simulink library "ude"  (Simulink 8.2)
settings: Solver=ode1  StartTime=0.0  StopTime=Inf  FixedStep=0.001  RelTol=1e-3
PostLoadFcn:
  | , if any(exist('dsrtsu_mdlpostloadfcn', 'file') == [2, 3, 6]), try dsrtsu_mdlpostloadfcn('Execute', bdroot); catch fprintf('Error in PostLoadFcn (dsrtsu_mdlpostloadfcn) for model "%s":\n %s\n', bdroot, lasterr); end, end,
undefined symbols (not defined in the file or in its folder): FALSE, TRUE
libraries: hcu_lib x4, simulink x2
(part 1 of 2)
settings Model: RequirementInfo="{}  %GIDa_987fab82_ea26_42c4_899d_f6cf30f28fd4"  DSRTSU_INTERNAL_RTI_VER=450  DSRTSU_INTERNAL_RTI_TYPE=rti1401  RTICANMMDATA=struct('GeneralSetupData',struct('modelroot','D:\ActiveSafetyDepartment\SVN\trunk\ADAS_Softwares\HTDragon\software\sw_development\arch\app\ude','generalsettings',struct('filesettings',struct('destfolder',struct('Name','RTICANMM_FILES','Check',1),'buildfolder',struct('Name','.','Check',1),'AbsDestfolder',struct('Name','D:\ActiveSafetyDepartment\SVN\trunk\ADAS_Softwares\HTDragon\software\sw_development\arch\app\ude\RTICANMM_FILES'),'AbsBuildfolder',struct('Name','D:\ActiveSafetyDepartment\SVN\trunk\ADAS_Softwares\HTDragon\software\sw_development\arch\app\ude'))),'options',struct('addpaths',1,'rmpaths',1,'addtrcexclusion',logical(1),'cannavigator',struct('checkmonitoring',0),'show_usrtrc',0,'use_usrtrc',0),'advanced',struct('options',[1 1 1 1 1 1 1 1 1 1 1 1 1 1 1 1 1 1 1 1 1 1 1 1 1 1 1 1 1 1 1 1 1 1 1 1 1 1 1 1 1 1 1 1 1 1 1 1 1 1 1 1 1 1 1 1 1 1 1 1 1 1 1 1 1 1 1 1 1 1 1 1 1 1 1 1 1 1 1 1 1 1 1 1 1 1 1 1 1 1 1 1 1 1 1 1 1 1 1 1]),'MPSetup',{{}},'modelname','ude','block','ude'))  DSRTSU_INTERNAL_RTIFPGA=40  Creator=11116  LastModifiedBy=14069

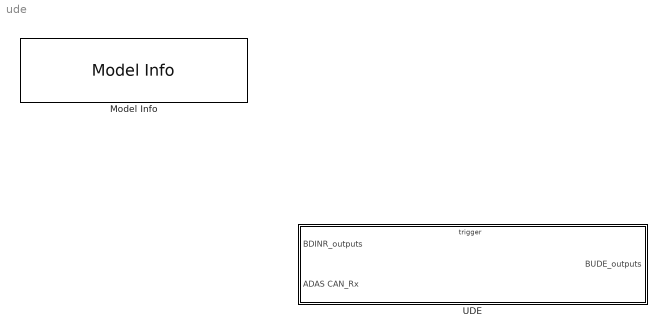
== system ude ==
  Model Info : simulink/Model-Wide Utilities/Model Info  InitialBlockCM=None  BlockCM=None  Frame=on  DisplayStringWithTags=|  HorizontalTextAlignment=Left  LeftAlignmentValue=0.02  SourceBlockDiagram=ude  TagMaxNumber=20
      | Model Version        : %<ModelVersion>
      | Creator                   : %<Creator>
      | Last Modified By    : %<LastModifiedBy>
  UDE : Subsystem
      settings: RTWSystemCode=Nonreusable function  RTWFcnNameOpts=Use subsystem name  RTWFileNameOpts=Use subsystem name

== system ude/UDE ==
  BDINR_outputs : Inport  OutDataTypeStr=Bus: BDINR_outputs
  ADAS CAN_Rx : Inport  Port=2
  trig_UDE : TriggerPort  TriggerType=function-call
  ude : Subsystem
  BUDE_outputs : Outport
  wires:
  ADAS CAN_Rx/1 -> ude/2(ADAS CAN_Rx)
  BDINR_outputs/1 -> ude/1(BDINR_outputs)
  ude/1(BUDE_outputs) -> BUDE_outputs/1

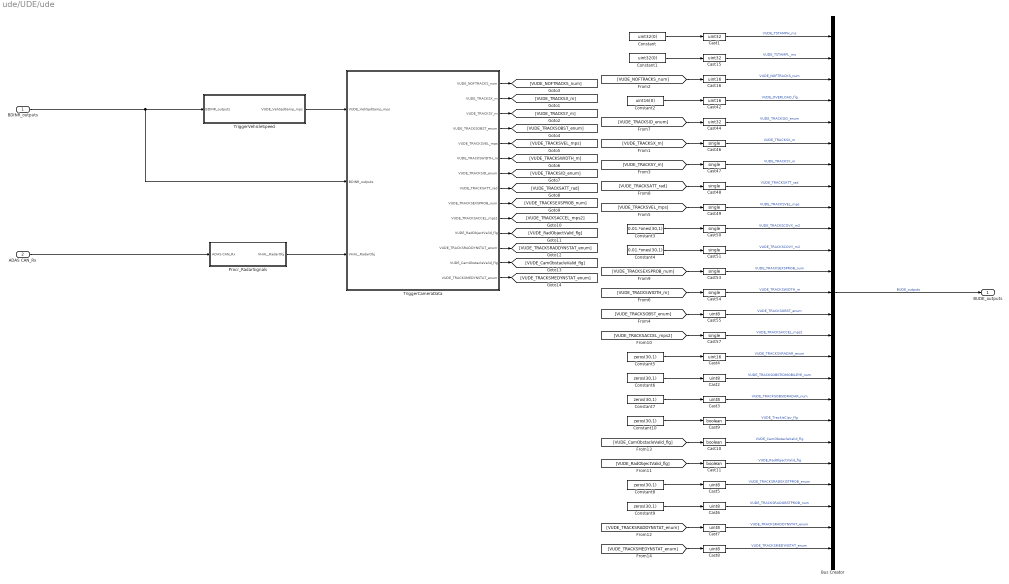
== system ude/UDE/ude ==
  BDINR_outputs : Inport
  ADAS CAN_Rx : Inport  Port=2
  Bus Creator : BusCreator  Inputs=25  OutDataTypeStr=Bus: BUDE_outputs
  Cast1 : DataTypeConversion  OutDataTypeStr=uint32  RndMeth=Zero
  Cast10 : DataTypeConversion  OutDataTypeStr=boolean  RndMeth=Zero
  Cast11 : DataTypeConversion  OutDataTypeStr=boolean  RndMeth=Zero
  Cast15 : DataTypeConversion  OutDataTypeStr=uint32  RndMeth=Zero
  Cast16 : DataTypeConversion  OutDataTypeStr=uint16  RndMeth=Zero
  Cast{2..3,5..8,55} (7 alike) : DataTypeConversion  OutDataTypeStr=uint8  RndMeth=Zero
  Cast4 : DataTypeConversion  OutDataTypeStr=uint16  RndMeth=Zero
  Cast42 : DataTypeConversion  OutDataTypeStr=uint16  RndMeth=Zero
  Cast44 : DataTypeConversion  OutDataTypeStr=uint32  RndMeth=Zero
  Cast{46..51,53..54,57} (9 alike) : DataTypeConversion  OutDataTypeStr=single  RndMeth=Zero
  Cast9 : DataTypeConversion  OutDataTypeStr=boolean  RndMeth=Zero
  Constant : Constant  Value=uint32(0)
  Constant1 : Constant  Value=uint32(0)
  Constant10 : Constant  Value=zeros(30,1)  OutDataTypeStr=boolean
  Constant2 : Constant  Value=uint16(0)
  Constant3 : Constant  Value=0.01.*ones(30,1)  OutDataTypeStr=single
  Constant4 : Constant  Value=0.01.*ones(30,1)  OutDataTypeStr=single
  Constant5 : Constant  Value=zeros(30,1)  OutDataTypeStr=uint16
  Constant{6..9} (4 alike) : Constant  Value=zeros(30,1)  OutDataTypeStr=uint8
  Procr_RadarSignals : Subsystem
  TriggerCameraData : Subsystem  TreatAsAtomicUnit=on
  TriggerVehicleSpeed : Subsystem  TreatAsAtomicUnit=on
  BUDE_outputs : Outport  OutDataTypeStr=Bus: BUDE_outputs
  wires:
  Constant9/1 -> Cast6/1
  Constant8/1 -> Cast5/1
  Constant7/1 -> Cast3/1
  Constant6/1 -> Cast2/1
  Constant5/1 -> Cast4/1
  Constant10/1 -> Cast9/1
  Constant4/1 -> Cast51/1
  Constant3/1 -> Cast50/1
  Constant2/1 -> Cast42/1
  [VUDE_CamObstacleValid_flg] -> Cast10/1
  [VUDE_TRACKSMEDYNSTAT_enum] -> Cast8/1
  [VUDE_TRACKSRADDYNSTAT_enum] -> Cast7/1
  [VUDE_RadObjectValid_flg] -> Cast11/1
  [VUDE_TRACKSACCEL_mps2] -> Cast57/1
  [VUDE_TRACKSEXSPROB_num] -> Cast53/1
  [VUDE_TRACKSATT_rad] -> Cast48/1
  [VUDE_TRACKSID_enum] -> Cast44/1
  [VUDE_TRACKSWIDTH_m] -> Cast54/1
  [VUDE_TRACKSVEL_mps] -> Cast49/1
  [VUDE_TRACKSOBST_enum] -> Cast55/1
  [VUDE_TRACKSY_m] -> Cast47/1
  [VUDE_TRACKSX_m] -> Cast46/1
  [VUDE_NOFTRACKS_num] -> Cast16/1
  TriggerCameraData/14(VUDE_TRACKSMEDYNSTAT_enum) -> [VUDE_TRACKSMEDYNSTAT_enum]
  TriggerCameraData/13(VUDE_CamObstacleValid_flg) -> [VUDE_CamObstacleValid_flg]
  TriggerCameraData/12(VUDE_TRACKSRADDYNSTAT_enum) -> [VUDE_TRACKSRADDYNSTAT_enum]
  TriggerCameraData/11(VUDE_RadObjectValid_flg) -> [VUDE_RadObjectValid_flg]
  TriggerCameraData/10(VUDE_TRACKSACCEL_mps2) -> [VUDE_TRACKSACCEL_mps2]
  TriggerCameraData/9(VUDE_TRACKSEXSPROB_num) -> [VUDE_TRACKSEXSPROB_num]
  TriggerCameraData/8(VUDE_TRACKSATT_rad) -> [VUDE_TRACKSATT_rad]
  TriggerCameraData/7(VUDE_TRACKSID_enum) -> [VUDE_TRACKSID_enum]
  TriggerCameraData/6(VUDE_TRACKSWIDTH_m) -> [VUDE_TRACKSWIDTH_m]
  TriggerCameraData/5(VUDE_TRACKSVEL_mps) -> [VUDE_TRACKSVEL_mps]
  TriggerCameraData/4(VUDE_TRACKSOBST_enum) -> [VUDE_TRACKSOBST_enum]
  TriggerCameraData/3(VUDE_TRACKSY_m) -> [VUDE_TRACKSY_m]
  TriggerCameraData/2(VUDE_TRACKSX_m) -> [VUDE_TRACKSX_m]
  TriggerCameraData/1(VUDE_NOFTRACKS_num) -> [VUDE_NOFTRACKS_num]
  Cast8/1 -> Bus Creator/25  "VUDE_TRACKSMEDYNSTAT_enum"
  Cast11/1 -> Bus Creator/21  "VUDE_RadObjectValid_flg"
  Cast10/1 -> Bus Creator/20  "VUDE_CamObstacleValid_flg"
  Cast9/1 -> Bus Creator/19  "VUDE_TrackIsCipv_flg"
  Cast7/1 -> Bus Creator/24  "VUDE_TRACKSRADDYNSTAT_enum"
  Cast6/1 -> Bus Creator/23  "VUDE_TRACKSRADOBSTPROB_num"
  Cast5/1 -> Bus Creator/22  "VUDE_TRACKSRADEXISTPROB_enum"
  Cast3/1 -> Bus Creator/18  "VUDE_TRACKSOBSIDRADAR_num"
  Cast2/1 -> Bus Creator/17  "VUDE_TRACKSOBSTIDMOBILEYE_num"
  Cast53/1 -> Bus Creator/12  "VUDE_TRACKSEXSPROB_num"
  Cast54/1 -> Bus Creator/13  "VUDE_TRACKSWIDTH_m"
  Cast55/1 -> Bus Creator/14  "VUDE_TRACKSOBST_enum"
  Cast57/1 -> Bus Creator/15  "VUDE_TRACKSACCEL_mps2"
  Cast51/1 -> Bus Creator/11  "VUDE_TRACKSCOVY_m2"
  Cast50/1 -> Bus Creator/10  "VUDE_TRACKSCOVX_m2"
  Cast49/1 -> Bus Creator/9  "VUDE_TRACKSVEL_mps"
  Cast48/1 -> Bus Creator/8  "VUDE_TRACKSATT_rad"
  Cast47/1 -> Bus Creator/7  "VUDE_TRACKSY_m"
  Cast46/1 -> Bus Creator/6  "VUDE_TRACKSX_m"
  Cast44/1 -> Bus Creator/5  "VUDE_TRACKSID_enum"
  Cast42/1 -> Bus Creator/4  "VUDE_OVERLOAD_flg"
  Cast16/1 -> Bus Creator/3  "VUDE_NOFTRACKS_num"
  Cast15/1 -> Bus Creator/2  "VUDE_TSTAMPL_ms"
  Cast1/1 -> Bus Creator/1  "VUDE_TSTAMPH_ms"
  Bus Creator/1 -> BUDE_outputs/1  "BUDE_outputs"
  Cast4/1 -> Bus Creator/16  "VUDE_TRACKSVRADAR_enum"
  Constant/1 -> Cast1/1
  Constant1/1 -> Cast15/1
  BDINR_outputs/1 -> TriggerCameraData/2(BDINR_outputs), TriggerVehicleSpeed/1(BDINR_outputs)
  TriggerVehicleSpeed/1(VUDE_VehSpdSamp_mps) -> TriggerCameraData/1(VUDE_VehSpdSamp_mps)
  Procr_RadarSignals/1(VHAL_RadarObj) -> TriggerCameraData/3(VHAL_RadarObj)
  ADAS CAN_Rx/1 -> Procr_RadarSignals/1(ADAS CAN_Rx)

== system ude/UDE/ude/Procr_RadarSignals ==
  ADAS CAN_Rx : Inport
  Bus Creator : BusCreator  Inputs=11
  Procr_RadarSignals : Subsystem
  VHAL_RadarObj : Outport
  wires:
  ADAS CAN_Rx/1 -> Procr_RadarSignals/1(ADAS CAN_Rx)
  Procr_RadarSignals/7(VHAL_RadarObjType10_enum_InProc) -> Bus Creator/7
  Procr_RadarSignals/5(VHAL_RadarObjVelX10_mps_InProc) -> Bus Creator/5
  Procr_RadarSignals/8(VHAL_RadarObjVelY10_mps_InProc) -> Bus Creator/8
  Procr_RadarSignals/3(VHAL_RadarObjPosX10_m_InProc) -> Bus Creator/3
  Procr_RadarSignals/9(VHAL_RadarObjAccX10_mps2_InProc) -> Bus Creator/9
  Procr_RadarSignals/4(VHAL_RadarObjPosY10_m_InProc) -> Bus Creator/4
  Procr_RadarSignals/2(VHAL_RadarObjID10_num_InProc) -> Bus Creator/2
  Procr_RadarSignals/6(VHAL_RadarObjStatus10_enum_InProc) -> Bus Creator/6
  Bus Creator/1 -> VHAL_RadarObj/1
  Procr_RadarSignals/1(VHAL_NoObj_num_InProc) -> Bus Creator/1
  Procr_RadarSignals/10(VHAL_RadarObjValid10_flg_InProc) -> Bus Creator/10
  Procr_RadarSignals/11(VHAL_RadarObjWidth10_m_InProc) -> Bus Creator/11

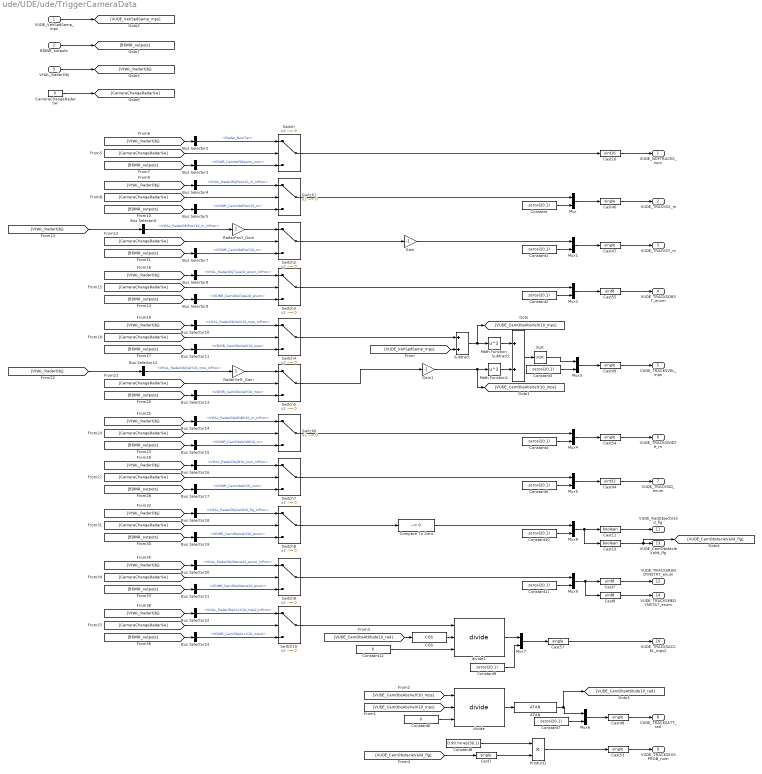
== system ude/UDE/ude/TriggerCameraData ==
  VUDE_VehSpdSamp_mps : Inport
  BDINR_outputs : Inport  Port=2
  VHAL_RadarObj : Inport  Port=3
  ATAN : hcu_lib/ATAN
  Bus Selector10 : BusSelector  OutputSignals=VHAL_RadarObjVelX10_mps_InProc
  Bus Selector11 : BusSelector  OutputSignals=VDINR_CamObsVelX10_mps
  Bus Selector12 : BusSelector  OutputSignals=VHAL_RadarObjVelY10_mps_InProc
  Bus Selector13 : BusSelector  OutputSignals=VDINR_CamObsVelY10_mps
  Bus Selector14 : BusSelector  OutputSignals=VHAL_RadarObjWidth10_m_InProc
  Bus Selector15 : BusSelector  OutputSignals=VDINR_CamObsWidth10_m
  Bus Selector16 : BusSelector  OutputSignals=VHAL_RadarObjID10_num_InProc
  Bus Selector17 : BusSelector  OutputSignals=VDINR_CamObsID10_num
  Bus Selector18 : BusSelector  OutputSignals=VHAL_RadarObjValid10_flg_InProc
  Bus Selector19 : BusSelector  OutputSignals=VDINR_CamObsValid10_enum
  Bus Selector2 : BusSelector  OutputSignals=Radar_NumTar
  Bus Selector20 : BusSelector  OutputSignals=VHAL_RadarObjStatus10_enum_InProc
  Bus Selector21 : BusSelector  OutputSignals=VDINR_CamObsStatus10_enum
  Bus Selector22 : BusSelector  OutputSignals=VHAL_RadarObjAccX10_mps2_InProc
  Bus Selector23 : BusSelector  OutputSignals=VDINR_CamObsAccX10_mps2
  Bus Selector3 : BusSelector  OutputSignals=VDINR_CamNofObjects_num
  Bus Selector4 : BusSelector  OutputSignals=VHAL_RadarObjPosX10_m_InProc
  Bus Selector5 : BusSelector  OutputSignals=VDINR_CamObsPosX10_m
  Bus Selector6 : BusSelector  OutputSignals=VHAL_RadarObjPosY10_m_InProc
  Bus Selector7 : BusSelector  OutputSignals=VDINR_CamObsPosY10_m
  Bus Selector8 : BusSelector  OutputSignals=VHAL_RadarObjType10_enum_InProc
  Bus Selector9 : BusSelector  OutputSignals=VDINR_CamObsType10_enum
  COS : hcu_lib/COS
  CameraChangeRadarSw : Constant  Value=0
  Cast{1,46..49,53..54,57} (8 alike) : DataTypeConversion  OutDataTypeStr=single  RndMeth=Zero
  Cast10 : DataTypeConversion  OutDataTypeStr=boolean  RndMeth=Zero
  Cast11 : DataTypeConversion  OutDataTypeStr=boolean  RndMeth=Zero
  Cast16 : DataTypeConversion  OutDataTypeStr=uint16  RndMeth=Zero
  Cast44 : DataTypeConversion  OutDataTypeStr=uint32  RndMeth=Zero
  Cast55 : DataTypeConversion  OutDataTypeStr=uint8  RndMeth=Zero
  Cast7 : DataTypeConversion  OutDataTypeStr=uint8  RndMeth=Zero
  Cast8 : DataTypeConversion  OutDataTypeStr=uint8  RndMeth=Zero
  Compare To Zero : simulink/Logic and Bit Operations/Compare To Zero  relop=~=  OutDataTypeStr=boolean
  Constant{,1,3..4,7,9} (6 alike) : Constant  Value=zeros(20,1)  OutDataTypeStr=single
  Constant10 : Constant  Value=zeros(20,1)  OutDataTypeStr=boolean
  Constant11 : Constant  Value=zeros(20,1)  OutDataTypeStr=uint8
  Constant12 : Constant  Value=0  OutDataTypeStr=single
  Constant2 : Constant  Value=zeros(20,1)  OutDataTypeStr=uint8
  Constant5 : Constant  Value=zeros(20,1)  OutDataTypeStr=uint8
  Constant6 : Constant  Value=0  OutDataTypeStr=single
  Constant8 : Constant  Value=0.99.*ones(30,1)  OutDataTypeStr=single
  Gain : Gain  Gain=-1
  Gain1 : Gain  Gain=-1
  Math Function : Math  Operator=square  SaturateOnIntegerOverflow=on
  Math Function1 : Math  Operator=square  SaturateOnIntegerOverflow=on
  Mux{,1..9} (10 alike) : Mux  Inputs=2
  Product1 : Product
  RadarPosY_Gain : Gain
  RadarVelY_Gain : Gain
  Sqrt : Sqrt  SaturateOnIntegerOverflow=on
  Subtract : Sum
  Subtract1 : Sum
  Switch{,1..10} (11 alike) : Switch  Criteria=u2 ~= 0
  divide : hcu_lib/divide
  divide1 : hcu_lib/divide
  VUDE_NOFTRACKS_num : Outport
  VUDE_TRACKSX_m : Outport  Port=2
  VUDE_TRACKSY_m : Outport  Port=3
  VUDE_TRACKSOBST_enum : Outport  Port=4
  VUDE_TRACKSVEL_mps : Outport  Port=5
  VUDE_TRACKSWIDTH_m : Outport  Port=6
  VUDE_TRACKSID_enum : Outport  Port=7
  VUDE_TRACKSATT_rad : Outport  Port=8
  VUDE_TRACKSEXSPROB_num : Outport  Port=9
  VUDE_TRACKSACCEL_mps2 : Outport  Port=10
  VUDE_RadObjectValid_flg : Outport  Port=11
  VUDE_TRACKSRADDYNSTAT_enum : Outport  Port=12
  VUDE_CamObstacleValid_flg : Outport  Port=13
  VUDE_TRACKSMEDYNSTAT_enum : Outport  Port=14
  wires:
  Constant12/1 -> divide1/3
  Cast1/1 -> Product1/2
  Constant8/1 -> Product1/1
  [VUDE_CamObstacleValid_flg] -> Cast1/1
  Mux9/1 -> Cast7/1, Cast8/1
  Constant11/1 -> Mux9/2
  Mux8/1 -> Cast11/1, Cast10/1
  Compare To Zero/1 -> Mux8/1
  Constant10/1 -> Mux8/2
  Constant9/1 -> Mux7/2
  Mux7/1 -> Cast57/1
  divide1/1 -> Mux7/1
  COS/1 -> divide1/2
  [VUDE_CamObsAttitude10_rad] -> COS/1
  ATAN/1 -> Mux6/1, [VUDE_CamObsAttitude10_rad]
  Product1/1 -> Cast53/1
  Mux6/1 -> Cast48/1
  Constant7/1 -> Mux6/2
  Constant6/1 -> divide/3
  divide/1 -> ATAN/1
  [VUDE_CamObsAbsVelY10_mps] -> divide/1
  [VUDE_CamObsAbsVelX10_mps] -> divide/2
  Gain1/1 -> Math Function1/1, [VUDE_CamObsAbsVelY10_mps]
  Mux5/1 -> Cast44/1
  Constant5/1 -> Mux5/2
  Mux4/1 -> Cast54/1
  Constant4/1 -> Mux4/2
  Mux3/1 -> Cast49/1
  Sqrt/1 -> Mux3/1
  Constant3/1 -> Mux3/2
  Subtract1/1 -> Sqrt/1
  Math Function1/1 -> Subtract1/2
  Math Function/1 -> Subtract1/1
  Subtract/1 -> Math Function/1, [VUDE_CamObsAbsVelX10_mps]
  [VUDE_VehSpdSamp_mps] -> Subtract/2
  VUDE_VehSpdSamp_mps/1 -> [VUDE_VehSpdSamp_mps]
  Gain/1 -> Mux1/1
  Mux2/1 -> Cast55/1
  Constant2/1 -> Mux2/2
  Mux1/1 -> Cast47/1
  Constant1/1 -> Mux1/2
  Constant/1 -> Mux/2
  Mux/1 -> Cast46/1
  Cast8/1 -> VUDE_TRACKSMEDYNSTAT_enum/1
  Cast10/1 -> VUDE_CamObstacleValid_flg/1, [VUDE_CamObstacleValid_flg]
  Cast7/1 -> VUDE_TRACKSRADDYNSTAT_enum/1
  Cast11/1 -> VUDE_RadObjectValid_flg/1
  Cast57/1 -> VUDE_TRACKSACCEL_mps2/1
  Cast53/1 -> VUDE_TRACKSEXSPROB_num/1
  Cast48/1 -> VUDE_TRACKSATT_rad/1
  Cast44/1 -> VUDE_TRACKSID_enum/1
  Cast54/1 -> VUDE_TRACKSWIDTH_m/1
  Cast49/1 -> VUDE_TRACKSVEL_mps/1
  Cast55/1 -> VUDE_TRACKSOBST_enum/1
  Cast47/1 -> VUDE_TRACKSY_m/1
  Cast46/1 -> VUDE_TRACKSX_m/1
  Cast16/1 -> VUDE_NOFTRACKS_num/1
  VHAL_RadarObj/1 -> [VHAL_RadarObj]
  CameraChangeRadarSw/1 -> [CameraChangeRadarSw]
  BDINR_outputs/1 -> [BDINR_outputs]
  Switch/1 -> Cast16/1
  [CameraChangeRadarSw] -> Switch/2
  [VHAL_RadarObj] -> Bus Selector2/1
  Bus Selector2/1 -> Switch/1  "<Radar_NumTar>"
  [BDINR_outputs] -> Bus Selector3/1
  Bus Selector3/1 -> Switch/3  "<VDINR_CamNofObjects_num>"
  Switch1/1 -> Mux/1
  [CameraChangeRadarSw] -> Switch1/2
  [VHAL_RadarObj] -> Bus Selector4/1
  Bus Selector4/1 -> Switch1/1  "<VHAL_RadarObjPosX10_m_InProc>"
  [BDINR_outputs] -> Bus Selector5/1
  Bus Selector5/1 -> Switch1/3  "<VDINR_CamObsPosX10_m>"
  [CameraChangeRadarSw] -> Switch2/2
  [VHAL_RadarObj] -> Bus Selector6/1
  Bus Selector6/1 -> RadarPosY_Gain/1  "<VHAL_RadarObjPosY10_m_InProc>"
  [BDINR_outputs] -> Bus Selector7/1
  Bus Selector7/1 -> Switch2/3  "<VDINR_CamObsPosY10_m>"
  Switch2/1 -> Gain/1
  RadarPosY_Gain/1 -> Switch2/1
  Switch3/1 -> Mux2/1
  [CameraChangeRadarSw] -> Switch3/2
  [VHAL_RadarObj] -> Bus Selector8/1
  Bus Selector8/1 -> Switch3/1  "<VHAL_RadarObjType10_enum_InProc>"
  [BDINR_outputs] -> Bus Selector9/1
  Bus Selector9/1 -> Switch3/3  "<VDINR_CamObsType10_enum>"
  Switch4/1 -> Subtract/1
  [CameraChangeRadarSw] -> Switch4/2
  [VHAL_RadarObj] -> Bus Selector10/1
  Bus Selector10/1 -> Switch4/1  "<VHAL_RadarObjVelX10_mps_InProc>"
  [BDINR_outputs] -> Bus Selector11/1
  Bus Selector11/1 -> Switch4/3  "<VDINR_CamObsVelX10_mps>"
  [CameraChangeRadarSw] -> Switch5/2
  [VHAL_RadarObj] -> Bus Selector12/1
  Bus Selector12/1 -> RadarVelY_Gain/1  "<VHAL_RadarObjVelY10_mps_InProc>"
  [BDINR_outputs] -> Bus Selector13/1
  Bus Selector13/1 -> Switch5/3  "<VDINR_CamObsVelY10_mps>"
  Switch5/1 -> Gain1/1
  RadarVelY_Gain/1 -> Switch5/1
  Switch6/1 -> Mux4/1
  [CameraChangeRadarSw] -> Switch6/2
  [VHAL_RadarObj] -> Bus Selector14/1
  Bus Selector14/1 -> Switch6/1  "<VHAL_RadarObjWidth10_m_InProc>"
  [BDINR_outputs] -> Bus Selector15/1
  Bus Selector15/1 -> Switch6/3  "<VDINR_CamObsWidth10_m>"
  Switch7/1 -> Mux5/1
  [CameraChangeRadarSw] -> Switch7/2
  [VHAL_RadarObj] -> Bus Selector16/1
  Bus Selector16/1 -> Switch7/1  "<VHAL_RadarObjID10_num_InProc>"
  [BDINR_outputs] -> Bus Selector17/1
  Bus Selector17/1 -> Switch7/3  "<VDINR_CamObsID10_num>"
  [CameraChangeRadarSw] -> Switch8/2
  [VHAL_RadarObj] -> Bus Selector18/1
  Bus Selector18/1 -> Switch8/1  "<VHAL_RadarObjValid10_flg_InProc>"
  [BDINR_outputs] -> Bus Selector19/1
  Bus Selector19/1 -> Switch8/3  "<VDINR_CamObsValid10_enum>"
  Switch8/1 -> Compare To Zero/1
  Switch9/1 -> Mux9/1
  [CameraChangeRadarSw] -> Switch9/2
  [VHAL_RadarObj] -> Bus Selector20/1
  Bus Selector20/1 -> Switch9/1  "<VHAL_RadarObjStatus10_enum_InProc>"
  [BDINR_outputs] -> Bus Selector21/1
  Bus Selector21/1 -> Switch9/3  "<VDINR_CamObsStatus10_enum>"
  Switch10/1 -> divide1/1
  [CameraChangeRadarSw] -> Switch10/2
  [VHAL_RadarObj] -> Bus Selector22/1
  Bus Selector22/1 -> Switch10/1  "<VHAL_RadarObjAccX10_mps2_InProc>"
  [BDINR_outputs] -> Bus Selector23/1
  Bus Selector23/1 -> Switch10/3  "<VDINR_CamObsAccX10_mps2>"

== system ude/UDE/ude/TriggerVehicleSpeed ==
  BDINR_outputs : Inport
  Bus Selector1 : BusSelector  OutputSignals=VDINR_VehSpd_mps
  Data Type Conversion : DataTypeConversion  OutDataTypeStr=single
  VUDE_VehSpdSamp_mps : Outport
  wires:
  Bus Selector1/1 -> Data Type Conversion/1  "<VDINR_VehSpd_mps>"
  BDINR_outputs/1 -> Bus Selector1/1
  Data Type Conversion/1 -> VUDE_VehSpdSamp_mps/1  "VUDE_VehSpdSamp_mps"

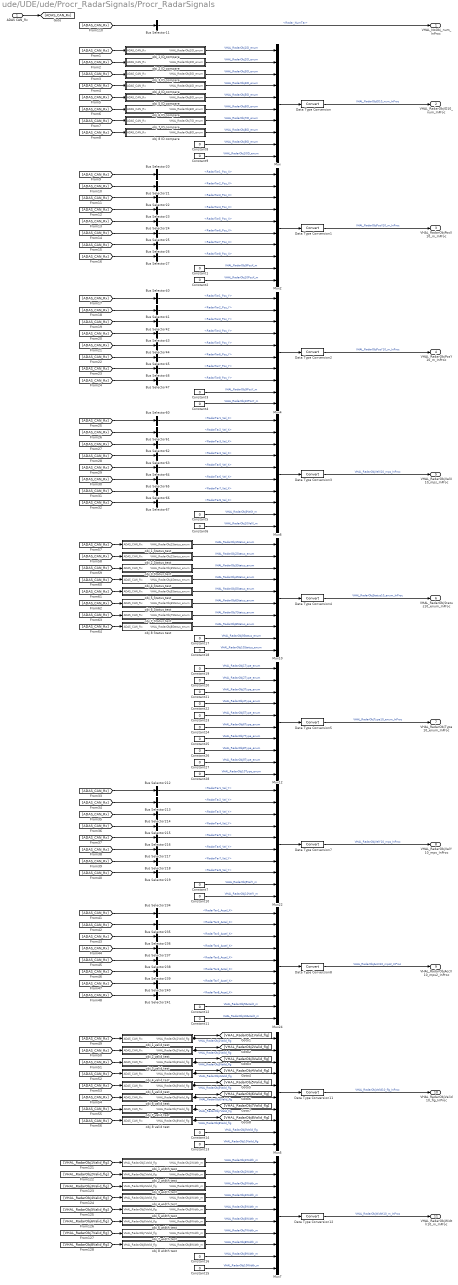
== system ude/UDE/ude/Procr_RadarSignals/Procr_RadarSignals ==
  ADAS CAN_Rx : Inport
  Bus Selector11 : BusSelector  OutputSignals=SENP45.Radar_NumTar
  Bus Selector20 : BusSelector  OutputSignals=SENP46.RadarTar1_Pos_X
  Bus Selector21 : BusSelector  OutputSignals=SENP48.RadarTar2_Pos_X
  Bus Selector212 : BusSelector  OutputSignals=SENP46.RadarTar1_Vel_Y
  Bus Selector213 : BusSelector  OutputSignals=SENP48.RadarTar2_Vel_Y
  Bus Selector214 : BusSelector  OutputSignals=SENP50.RadarTar3_Vel_Y
  Bus Selector215 : BusSelector  OutputSignals=SENP52.RadarTar4_Vel_Y
  Bus Selector216 : BusSelector  OutputSignals=SENP54.RadarTar5_Vel_Y
  Bus Selector217 : BusSelector  OutputSignals=SENP56.RadarTar6_Vel_Y
  Bus Selector218 : BusSelector  OutputSignals=SENP58.RadarTar7_Vel_Y
  Bus Selector219 : BusSelector  OutputSignals=SENP60.RadarTar8_Vel_Y
  Bus Selector22 : BusSelector  OutputSignals=SENP50.RadarTar3_Pos_X
  Bus Selector23 : BusSelector  OutputSignals=SENP52.RadarTar4_Pos_X
  Bus Selector234 : BusSelector  OutputSignals=SENP47.RadarTar1_Accel_X
  Bus Selector235 : BusSelector  OutputSignals=SENP49.RadarTar2_Accel_X
  Bus Selector236 : BusSelector  OutputSignals=SENP51.RadarTar3_Accel_X
  Bus Selector237 : BusSelector  OutputSignals=SENP53.RadarTar4_Accel_X
  Bus Selector238 : BusSelector  OutputSignals=SENP55.RadarTar5_Accel_X
  Bus Selector239 : BusSelector  OutputSignals=SENP57.RadarTar6_Accel_X
  Bus Selector24 : BusSelector  OutputSignals=SENP54.RadarTar5_Pos_X
  Bus Selector240 : BusSelector  OutputSignals=SENP59.RadarTar7_Accel_X
  Bus Selector241 : BusSelector  OutputSignals=SENP61.RadarTar8_Accel_X
  Bus Selector25 : BusSelector  OutputSignals=SENP56.RadarTar6_Pos_X
  Bus Selector26 : BusSelector  OutputSignals=SENP58.RadarTar7_Pos_X
  Bus Selector27 : BusSelector  OutputSignals=SENP60.RadarTar8_Pos_X
  Bus Selector40 : BusSelector  OutputSignals=SENP46.RadarTar1_Pos_Y
  Bus Selector41 : BusSelector  OutputSignals=SENP48.RadarTar2_Pos_Y
  Bus Selector42 : BusSelector  OutputSignals=SENP50.RadarTar3_Pos_Y
  Bus Selector43 : BusSelector  OutputSignals=SENP52.RadarTar4_Pos_Y
  Bus Selector44 : BusSelector  OutputSignals=SENP54.RadarTar5_Pos_Y
  Bus Selector45 : BusSelector  OutputSignals=SENP56.RadarTar6_Pos_Y
  Bus Selector46 : BusSelector  OutputSignals=SENP58.RadarTar7_Pos_Y
  Bus Selector47 : BusSelector  OutputSignals=SENP60.RadarTar8_Pos_Y
  Bus Selector60 : BusSelector  OutputSignals=SENP46.RadarTar1_Vel_X
  Bus Selector61 : BusSelector  OutputSignals=SENP48.RadarTar2_Vel_X
  Bus Selector62 : BusSelector  OutputSignals=SENP50.RadarTar3_Vel_X
  Bus Selector63 : BusSelector  OutputSignals=SENP52.RadarTar4_Vel_X
  Bus Selector64 : BusSelector  OutputSignals=SENP54.RadarTar5_Vel_X
  Bus Selector65 : BusSelector  OutputSignals=SENP56.RadarTar6_Vel_X
  Bus Selector66 : BusSelector  OutputSignals=SENP58.RadarTar7_Vel_X
  Bus Selector67 : BusSelector  OutputSignals=SENP60.RadarTar8_Vel_X
  Constant{1..12,15..28} (26 alike) : Constant  Value=0
  Constant13 : Constant  Value=0  OutDataTypeStr=boolean
  Constant14 : Constant  Value=0  OutDataTypeStr=boolean
  Data Type Conversion{,1..5,7..8,11..12} (10 alike) : DataTypeConversion
  Mux{,2,4..7,10,12,22,24} (10 alike) : Mux  Inputs=10
  obj 1 ID compare : Subsystem
  obj 1 Status test : Subsystem
  obj 1 valid test : Subsystem
  obj 1 width test : Subsystem
  obj 2 ID compare : Subsystem
  obj 2 Status test : Subsystem
  obj 2 valid test : Subsystem
  obj 2 width test : Subsystem
  obj 3 ID compare : Subsystem
  obj 3 Status test : Subsystem
  obj 3 valid test : Subsystem
  obj 3 width test : Subsystem
  obj 4 ID compare : Subsystem
  obj 4 Status test : Subsystem
  obj 4 valid test : Subsystem
  obj 4 width test : Subsystem
  obj 5 ID compare : Subsystem
  obj 5 Status test : Subsystem
  obj 5 valid test : Subsystem
  obj 5 width test : Subsystem
  obj 6 ID compare : Subsystem
  obj 6 Status test : Subsystem
  obj 6 valid test : Subsystem
  obj 6 width test : Subsystem
  obj 7 ID compare : Subsystem
  obj 7 Status test : Subsystem
  obj 7 valid test : Subsystem
  obj 7 width test : Subsystem
  obj 8 ID compare : Subsystem
  obj 8 Status test : Subsystem
  obj 8 valid test : Subsystem
  obj 8 width test : Subsystem
  VHAL_NoObj_num_InProc : Outport
  VHAL_RadarObjID10_num_InProc : Outport  Port=2
  VHAL_RadarObjPosX10_m_InProc : Outport  Port=3
  VHAL_RadarObjPosY10_m_InProc : Outport  Port=4
  VHAL_RadarObjVelX10_mps_InProc : Outport  Port=5
  VHAL_RadarObjStatus10_enum_InProc : Outport  Port=6
  VHAL_RadarObjType10_enum_InProc : Outport  Port=7
  VHAL_RadarObjVelY10_mps_InProc : Outport  Port=8
  VHAL_RadarObjAccX10_mps2_InProc : Outport  Port=9
  VHAL_RadarObjValid10_flg_InProc : Outport  Port=10
  VHAL_RadarObjWidth10_m_InProc : Outport  Port=11
  wires:
  ADAS CAN_Rx/1 -> [ADAS_CAN_Rx]
  Data Type Conversion/1 -> VHAL_RadarObjID10_num_InProc/1  "VHAL_RadarObjID10_num_InProc"
  Bus Selector20/1 -> Mux2/1  "<RadarTar1_Pos_X>"
  Bus Selector21/1 -> Mux2/2  "<RadarTar2_Pos_X>"
  Bus Selector22/1 -> Mux2/3  "<RadarTar3_Pos_X>"
  Bus Selector23/1 -> Mux2/4  "<RadarTar4_Pos_X>"
  Bus Selector24/1 -> Mux2/5  "<RadarTar5_Pos_X>"
  Bus Selector25/1 -> Mux2/6  "<RadarTar6_Pos_X>"
  Bus Selector26/1 -> Mux2/7  "<RadarTar7_Pos_X>"
  Bus Selector27/1 -> Mux2/8  "<RadarTar8_Pos_X>"
  [ADAS_CAN_Rx] -> Bus Selector20/1
  [ADAS_CAN_Rx] -> Bus Selector21/1
  [ADAS_CAN_Rx] -> Bus Selector22/1
  [ADAS_CAN_Rx] -> Bus Selector23/1
  [ADAS_CAN_Rx] -> Bus Selector24/1
  [ADAS_CAN_Rx] -> Bus Selector25/1
  [ADAS_CAN_Rx] -> Bus Selector26/1
  [ADAS_CAN_Rx] -> Bus Selector27/1
  Mux2/1 -> Data Type Conversion1/1
  Bus Selector40/1 -> Mux4/1  "<RadarTar1_Pos_Y>"
  Bus Selector41/1 -> Mux4/2  "<RadarTar2_Pos_Y>"
  Bus Selector42/1 -> Mux4/3  "<RadarTar3_Pos_Y>"
  Bus Selector43/1 -> Mux4/4  "<RadarTar4_Pos_Y>"
  Bus Selector44/1 -> Mux4/5  "<RadarTar5_Pos_Y>"
  Bus Selector45/1 -> Mux4/6  "<RadarTar6_Pos_Y>"
  Bus Selector46/1 -> Mux4/7  "<RadarTar7_Pos_Y>"
  Bus Selector47/1 -> Mux4/8  "<RadarTar8_Pos_Y>"
  Mux4/1 -> Data Type Conversion2/1
  Bus Selector60/1 -> Mux6/1  "<RadarTar1_Vel_X>"
  Bus Selector61/1 -> Mux6/2  "<RadarTar2_Vel_X>"
  Bus Selector62/1 -> Mux6/3  "<RadarTar3_Vel_X>"
  Bus Selector63/1 -> Mux6/4  "<RadarTar4_Vel_X>"
  Bus Selector64/1 -> Mux6/5  "<RadarTar5_Vel_X>"
  Bus Selector65/1 -> Mux6/6  "<RadarTar6_Vel_X>"
  Bus Selector66/1 -> Mux6/7  "<RadarTar7_Vel_X>"
  Bus Selector67/1 -> Mux6/8  "<RadarTar8_Vel_X>"
  Mux6/1 -> Data Type Conversion3/1
  Mux10/1 -> Data Type Conversion4/1
  Mux12/1 -> Data Type Conversion5/1
  [ADAS_CAN_Rx] -> obj 1 ID compare/1(ADAS_CAN_Rx)
  obj 1 ID compare/1(VHAL_RadarObj1ID_enum) -> Mux/1  "VHAL_RadarObj1ID_enum"
  obj 2 ID compare/1(VHAL_RadarObj2ID_enum) -> Mux/2  "VHAL_RadarObj2ID_enum"
  obj 3 ID compare/1(VHAL_RadarObj3ID_enum) -> Mux/3  "VHAL_RadarObj3ID_enum"
  obj 4 ID compare/1(VHAL_RadarObj4ID_enum) -> Mux/4  "VHAL_RadarObj4ID_enum"
  obj 5 ID compare/1(VHAL_RadarObj5ID_enum) -> Mux/5  "VHAL_RadarObj5ID_enum"
  obj 6 ID compare/1(VHAL_RadarObj6ID_enum) -> Mux/6  "VHAL_RadarObj6ID_enum"
  [ADAS_CAN_Rx] -> obj 2 ID compare/1(ADAS_CAN_Rx)
  [ADAS_CAN_Rx] -> obj 3 ID compare/1(ADAS_CAN_Rx)
  [ADAS_CAN_Rx] -> obj 4 ID compare/1(ADAS_CAN_Rx)
  [ADAS_CAN_Rx] -> obj 5 ID compare/1(ADAS_CAN_Rx)
  [ADAS_CAN_Rx] -> obj 6 ID compare/1(ADAS_CAN_Rx)
  [ADAS_CAN_Rx] -> obj 7 ID compare/1(ADAS_CAN_Rx)
  obj 7 ID compare/1(VHAL_RadarObj7ID_enum) -> Mux/7  "VHAL_RadarObj7ID_enum"
  obj 8 ID compare/1(VHAL_RadarObj8ID_enum) -> Mux/8  "VHAL_RadarObj8ID_enum"
  Constant8/1 -> Mux/9  "VHAL_RadarObj9ID_enum"
  Constant9/1 -> Mux/10  "VHAL_RadarObj10ID_enum"
  [ADAS_CAN_Rx] -> obj 8 ID compare/1(ADAS_CAN_Rx)
  [ADAS_CAN_Rx] -> Bus Selector40/1
  [ADAS_CAN_Rx] -> Bus Selector41/1
  [ADAS_CAN_Rx] -> Bus Selector42/1
  [ADAS_CAN_Rx] -> Bus Selector43/1
  [ADAS_CAN_Rx] -> Bus Selector44/1
  [ADAS_CAN_Rx] -> Bus Selector45/1
  [ADAS_CAN_Rx] -> Bus Selector46/1
  [ADAS_CAN_Rx] -> Bus Selector47/1
  [ADAS_CAN_Rx] -> Bus Selector60/1
  [ADAS_CAN_Rx] -> Bus Selector61/1
  [ADAS_CAN_Rx] -> Bus Selector62/1
  [ADAS_CAN_Rx] -> Bus Selector63/1
  [ADAS_CAN_Rx] -> Bus Selector64/1
  [ADAS_CAN_Rx] -> Bus Selector65/1
  [ADAS_CAN_Rx] -> Bus Selector66/1
  [ADAS_CAN_Rx] -> Bus Selector67/1
  Bus Selector212/1 -> Mux22/1  "<RadarTar1_Vel_Y>"
  Bus Selector213/1 -> Mux22/2  "<RadarTar2_Vel_Y>"
  Bus Selector214/1 -> Mux22/3  "<RadarTar3_Vel_Y>"
  Bus Selector215/1 -> Mux22/4  "<RadarTar4_Vel_Y>"
  Bus Selector216/1 -> Mux22/5  "<RadarTar5_Vel_Y>"
  Bus Selector217/1 -> Mux22/6  "<RadarTar6_Vel_Y>"
  Bus Selector218/1 -> Mux22/7  "<RadarTar7_Vel_Y>"
  Bus Selector219/1 -> Mux22/8  "<RadarTar8_Vel_Y>"
  [ADAS_CAN_Rx] -> Bus Selector212/1
  [ADAS_CAN_Rx] -> Bus Selector213/1
  [ADAS_CAN_Rx] -> Bus Selector214/1
  [ADAS_CAN_Rx] -> Bus Selector215/1
  [ADAS_CAN_Rx] -> Bus Selector216/1
  [ADAS_CAN_Rx] -> Bus Selector217/1
  [ADAS_CAN_Rx] -> Bus Selector218/1
  [ADAS_CAN_Rx] -> Bus Selector219/1
  Mux22/1 -> Data Type Conversion7/1
  Bus Selector234/1 -> Mux24/1  "<RadarTar1_Accel_X>"
  Bus Selector235/1 -> Mux24/2  "<RadarTar2_Accel_X>"
  Bus Selector236/1 -> Mux24/3  "<RadarTar3_Accel_X>"
  Bus Selector237/1 -> Mux24/4  "<RadarTar4_Accel_X>"
  Bus Selector238/1 -> Mux24/5  "<RadarTar5_Accel_X>"
  Bus Selector239/1 -> Mux24/6  "<RadarTar6_Accel_X>"
  Bus Selector240/1 -> Mux24/7  "<RadarTar7_Accel_X>"
  Bus Selector241/1 -> Mux24/8  "<RadarTar8_Accel_X>"
  [ADAS_CAN_Rx] -> Bus Selector234/1
  [ADAS_CAN_Rx] -> Bus Selector235/1
  [ADAS_CAN_Rx] -> Bus Selector236/1
  [ADAS_CAN_Rx] -> Bus Selector237/1
  [ADAS_CAN_Rx] -> Bus Selector238/1
  [ADAS_CAN_Rx] -> Bus Selector239/1
  [ADAS_CAN_Rx] -> Bus Selector240/1
  [ADAS_CAN_Rx] -> Bus Selector241/1
  Mux24/1 -> Data Type Conversion8/1
  [ADAS_CAN_Rx] -> Bus Selector11/1
  Bus Selector11/1 -> VHAL_NoObj_num_InProc/1  "<Radar_NumTar>"
  Mux5/1 -> Data Type Conversion11/1
  [ADAS_CAN_Rx] -> obj 1 valid test/1(ADAS_CAN_Rx)
  obj 1 valid test/1(VHAL_RadarObj1Valid_flg) -> Mux5/1, [VHAL_RadarObj1Valid_flg]  "VHAL_RadarObj1Valid_flg"
  [ADAS_CAN_Rx] -> obj 2 valid test/1(ADAS_CAN_Rx)
  [ADAS_CAN_Rx] -> obj 3 valid test/1(ADAS_CAN_Rx)
  obj 3 valid test/1(VHAL_RadarObj3Valid_flg) -> [VHAL_RadarObj3Valid_flg], Mux5/3  "VHAL_RadarObj3Valid_flg"
  [ADAS_CAN_Rx] -> obj 4 valid test/1(ADAS_CAN_Rx)
  obj 4 valid test/1(VHAL_RadarObj4Valid_flg) -> [VHAL_RadarObj4Valid_flg], Mux5/4  "VHAL_RadarObj4Valid_flg"
  [ADAS_CAN_Rx] -> obj 5 valid test/1(ADAS_CAN_Rx)
  obj 5 valid test/1(VHAL_RadarObj5Valid_flg) -> [VHAL_RadarObj5Valid_flg], Mux5/5  "VHAL_RadarObj5Valid_flg"
  [ADAS_CAN_Rx] -> obj 6 valid test/1(ADAS_CAN_Rx)
  obj 6 valid test/1(VHAL_RadarObj6Valid_flg) -> [VHAL_RadarObj6Valid_flg], Mux5/6  "VHAL_RadarObj6Valid_flg"
  [ADAS_CAN_Rx] -> obj 7 valid test/1(ADAS_CAN_Rx)
  obj 7 valid test/1(VHAL_RadarObj7Valid_flg) -> [VHAL_RadarObj7Valid_flg], Mux5/7  "VHAL_RadarObj7Valid_flg"
  [ADAS_CAN_Rx] -> obj 8 valid test/1(ADAS_CAN_Rx)
  obj 8 valid test/1(VHAL_RadarObj8Valid_flg) -> [VHAL_RadarObj8Valid_flg], Mux5/8  "VHAL_RadarObj8Valid_flg"
  obj 2 valid test/1(VHAL_RadarObj2Valid_flg) -> [VHAL_RadarObj2Valid_flg], Mux5/2  "VHAL_RadarObj1Valid_flg"
  Mux7/1 -> Data Type Conversion12/1
  [VHAL_RadarObj1Valid_flg] -> obj 1 width test/1(VHAL_RadarObj1Valid_flg)
  obj 1 width test/1(VHAL_RadarObj1Width_m) -> Mux7/1  "VHAL_RadarObj1Width_m"
  [VHAL_RadarObj2Valid_flg] -> obj 2 width test/1(VHAL_RadarObj2Valid_flg)
  obj 2 width test/1(VHAL_RadarObj2Width_m) -> Mux7/2  "VHAL_RadarObj2Width_m"
  [VHAL_RadarObj3Valid_flg] -> obj 3 width test/1(VHAL_RadarObj3Valid_flg)
  obj 3 width test/1(VHAL_RadarObj3Width_m) -> Mux7/3  "VHAL_RadarObj3Width_m"
  [VHAL_RadarObj4Valid_flg] -> obj 4 width test/1(VHAL_RadarObj4Valid_flg)
  obj 4 width test/1(VHAL_RadarObj4Width_m) -> Mux7/4  "VHAL_RadarObj4Width_m"
  [VHAL_RadarObj5Valid_flg] -> obj 5 width test/1(VHAL_RadarObj5Valid_flg)
  obj 5 width test/1(VHAL_RadarObj5Width_m) -> Mux7/5  "VHAL_RadarObj5Width_m"
  [VHAL_RadarObj6Valid_flg] -> obj 6 width test/1(VHAL_RadarObj6Valid_flg)
  obj 6 width test/1(VHAL_RadarObj6Width_m) -> Mux7/6  "VHAL_RadarObj6Width_m"
  [VHAL_RadarObj7Valid_flg] -> obj 7 width test/1(VHAL_RadarObj7Valid_flg)
  obj 7 width test/1(VHAL_RadarObj7Width_m) -> Mux7/7  "VHAL_RadarObj7Width_m"
  [VHAL_RadarObj8Valid_flg] -> obj 8 width test/1(VHAL_RadarObj8Valid_flg)
  obj 8 width test/1(VHAL_RadarObj8Width_m) -> Mux7/8  "VHAL_RadarObj8Width_m"
  Mux/1 -> Data Type Conversion/1
  Data Type Conversion1/1 -> VHAL_RadarObjPosX10_m_InProc/1  "VHAL_RadarObjPosX10_m_InProc"
  Data Type Conversion2/1 -> VHAL_RadarObjPosY10_m_InProc/1  "VHAL_RadarObjPosY10_m_InProc"
  Data Type Conversion3/1 -> VHAL_RadarObjVelX10_mps_InProc/1  "VHAL_RadarObjVelX10_mps_InProc"
  Data Type Conversion4/1 -> VHAL_RadarObjStatus10_enum_InProc/1  "VHAL_RadarObjStatus10_enum_InProc"
  Data Type Conversion5/1 -> VHAL_RadarObjType10_enum_InProc/1  "VHAL_RadarObjType10_enum_InProc"
  Data Type Conversion7/1 -> VHAL_RadarObjVelY10_mps_InProc/1  "VHAL_RadarObjVelY10_mps_InProc"
  Data Type Conversion8/1 -> VHAL_RadarObjAccX10_mps2_InProc/1  "VHAL_RadarObjAccX10_mps2_InProc"
  Data Type Conversion11/1 -> VHAL_RadarObjValid10_flg_InProc/1  "VHAL_RadarObjValid10_flg_InProc"
  Data Type Conversion12/1 -> VHAL_RadarObjWidth10_m_InProc/1  "VHAL_RadarObjWidth10_m_InProc"
  Constant1/1 -> Mux2/9  "VHAL_RadarObj9PosX_m"
  Constant2/1 -> Mux2/10  "VHAL_RadarObj10PosX_m"
  Constant3/1 -> Mux4/9  "VHAL_RadarObj9PosY_m"
  Constant4/1 -> Mux4/10  "VHAL_RadarObj10PosY_m"
  Constant5/1 -> Mux6/9  "VHAL_RadarObj9VelX_m"
  Constant6/1 -> Mux6/10  "VHAL_RadarObj10VelX_m"
  Constant7/1 -> Mux22/9  "VHAL_RadarObj9VelY_m"
  Constant10/1 -> Mux22/10  "VHAL_RadarObj10VelY_m"
  Constant12/1 -> Mux24/9  "VHAL_RadarObj9AccelX_m"
  Constant11/1 -> Mux24/10  "VHAL_RadarObj10AccelX_m"
  Constant14/1 -> Mux5/9  "VHAL_RadarObj9Valid_flg"
  Constant13/1 -> Mux5/10  "VHAL_RadarObj10Valid_flg"
  Constant16/1 -> Mux7/9  "VHAL_RadarObj9Width_m"
  Constant15/1 -> Mux7/10  "VHAL_RadarObj10Width_m"
  obj 1 Status test/1(VHAL_RadarObj1Status_enum) -> Mux10/1  "VHAL_RadarObj1Status_enum"
  [ADAS_CAN_Rx] -> obj 1 Status test/1(ADAS_CAN_Rx)
  obj 2 Status test/1(VHAL_RadarObj2Status_enum) -> Mux10/2  "VHAL_RadarObj2Status_enum"
  [ADAS_CAN_Rx] -> obj 2 Status test/1(ADAS_CAN_Rx)
  obj 3 Status test/1(VHAL_RadarObj3Status_enum) -> Mux10/3  "VHAL_RadarObj3Status_enum"
  [ADAS_CAN_Rx] -> obj 3 Status test/1(ADAS_CAN_Rx)
  Constant17/1 -> Mux10/9  "VHAL_RadarObj9Status_enum"
  Constant18/1 -> Mux10/10  "VHAL_RadarObj10Status_enum"
  obj 4 Status test/1(VHAL_RadarObj4Status_enum) -> Mux10/4  "VHAL_RadarObj4Status_enum"
  [ADAS_CAN_Rx] -> obj 4 Status test/1(ADAS_CAN_Rx)
  obj 5 Status test/1(VHAL_RadarObj5Status_enum) -> Mux10/5  "VHAL_RadarObj5Status_enum"
  [ADAS_CAN_Rx] -> obj 5 Status test/1(ADAS_CAN_Rx)
  obj 6 Status test/1(VHAL_RadarObj6Status_enum) -> Mux10/6  "VHAL_RadarObj6Status_enum"
  [ADAS_CAN_Rx] -> obj 6 Status test/1(ADAS_CAN_Rx)
  obj 7 Status test/1(VHAL_RadarObj7Status_enum) -> Mux10/7  "VHAL_RadarObj7Status_enum"
  [ADAS_CAN_Rx] -> obj 7 Status test/1(ADAS_CAN_Rx)
  obj 8 Status test/1(VHAL_RadarObj8Status_enum) -> Mux10/8  "VHAL_RadarObj8Status_enum"
  [ADAS_CAN_Rx] -> obj 8 Status test/1(ADAS_CAN_Rx)
  Constant19/1 -> Mux12/1  "VHAL_RadarObj1Type_enum"
  Constant20/1 -> Mux12/2  "VHAL_RadarObj2Type_enum"
  Constant21/1 -> Mux12/3  "VHAL_RadarObj3Type_enum"
  Constant22/1 -> Mux12/4  "VHAL_RadarObj4Type_enum"
  Constant23/1 -> Mux12/5  "VHAL_RadarObj5Type_enum"
  Constant24/1 -> Mux12/6  "VHAL_RadarObj6Type_enum"
  Constant25/1 -> Mux12/7  "VHAL_RadarObj7Type_enum"
  Constant26/1 -> Mux12/8  "VHAL_RadarObj8Type_enum"
  Constant27/1 -> Mux12/9  "VHAL_RadarObj9Type_enum"
  Constant28/1 -> Mux12/10  "VHAL_RadarObj10Type_enum"

== system ude/UDE/ude/Procr_RadarSignals/Procr_RadarSignals/obj 1 ID compare ==
  ADAS_CAN_Rx : Inport
  Bus Selector1 : BusSelector  OutputSignals=SENP46.RadarTar1_ID_A,SENP47.RadarTar1_ID_B
  Constant : Constant  Value=0
  Relational Operator : RelationalOperator  Operator===  OutDataTypeStr=boolean
  Switch : Switch  Criteria=u2 ~= 0
  VHAL_RadarObj1ID_enum : Outport
  wires:
  Bus Selector1/2 -> Relational Operator/2  "<RadarTar1_ID_B>"
  Bus Selector1/1 -> Switch/1, Relational Operator/1  "<RadarTar1_ID_A>"
  ADAS_CAN_Rx/1 -> Bus Selector1/1
  Switch/1 -> VHAL_RadarObj1ID_enum/1
  Relational Operator/1 -> Switch/2
  Constant/1 -> Switch/3

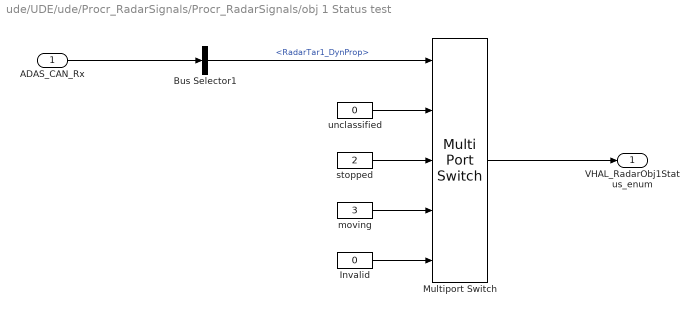
== system ude/UDE/ude/Procr_RadarSignals/Procr_RadarSignals/obj 1 Status test ==
  ADAS_CAN_Rx : Inport
  Bus Selector1 : BusSelector  OutputSignals=SENP47.RadarTar1_DynProp
  Invalid : Constant  Value=0
  Multiport Switch : MultiPortSwitch  DataPortOrder=Zero-based contiguous  Inputs=4
  moving : Constant  Value=3
  stopped : Constant  Value=2
  unclassified : Constant  Value=0
  VHAL_RadarObj1Status_enum : Outport
  wires:
  Multiport Switch/1 -> VHAL_RadarObj1Status_enum/1
  Invalid/1 -> Multiport Switch/5
  moving/1 -> Multiport Switch/4
  stopped/1 -> Multiport Switch/3
  unclassified/1 -> Multiport Switch/2
  Bus Selector1/1 -> Multiport Switch/1  "<RadarTar1_DynProp>"
  ADAS_CAN_Rx/1 -> Bus Selector1/1

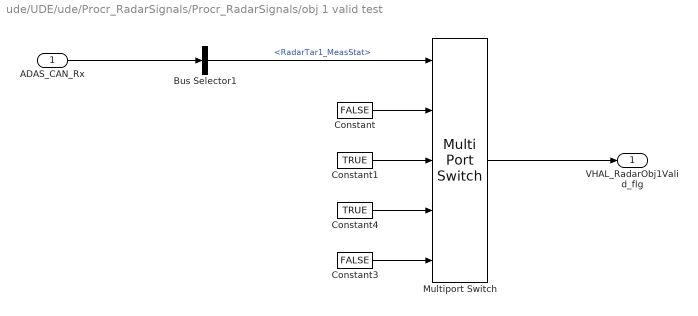
== system ude/UDE/ude/Procr_RadarSignals/Procr_RadarSignals/obj 1 valid test ==
  ADAS_CAN_Rx : Inport
  Bus Selector1 : BusSelector  OutputSignals=SENP47.RadarTar1_MeasStat
  Constant : Constant  Value=FALSE
  Constant1 : Constant  Value=TRUE
  Constant3 : Constant  Value=FALSE
  Constant4 : Constant  Value=TRUE
  Multiport Switch : MultiPortSwitch  DataPortOrder=Zero-based contiguous  Inputs=4
  VHAL_RadarObj1Valid_flg : Outport
  wires:
  Multiport Switch/1 -> VHAL_RadarObj1Valid_flg/1
  Constant3/1 -> Multiport Switch/5
  Constant4/1 -> Multiport Switch/4
  Constant1/1 -> Multiport Switch/3
  Constant/1 -> Multiport Switch/2
  Bus Selector1/1 -> Multiport Switch/1  "<RadarTar1_MeasStat>"
  ADAS_CAN_Rx/1 -> Bus Selector1/1

== system ude/UDE/ude/Procr_RadarSignals/Procr_RadarSignals/obj 1 width test ==
  VHAL_RadarObj1Valid_flg : Inport
  Constant : Constant  Value=0
  Constant1 : Constant  Value=2
  Multiport Switch : MultiPortSwitch  DataPortOrder=Zero-based contiguous  Inputs=2
  VHAL_RadarObj1Width_m : Outport
  wires:
  Multiport Switch/1 -> VHAL_RadarObj1Width_m/1
  Constant1/1 -> Multiport Switch/3
  Constant/1 -> Multiport Switch/2
  VHAL_RadarObj1Valid_flg/1 -> Multiport Switch/1

== system ude/UDE/ude/Procr_RadarSignals/Procr_RadarSignals/obj 2 ID compare ==
  ADAS_CAN_Rx : Inport
  Bus Selector1 : BusSelector  OutputSignals=SENP48.RadarTar2_ID_A,SENP49.RadarTar2_ID_B
  Constant : Constant  Value=0
  Relational Operator : RelationalOperator  Operator===  OutDataTypeStr=boolean
  Switch : Switch  Criteria=u2 ~= 0
  VHAL_RadarObj2ID_enum : Outport
  wires:
  Constant/1 -> Switch/3
  Relational Operator/1 -> Switch/2
  Switch/1 -> VHAL_RadarObj2ID_enum/1
  ADAS_CAN_Rx/1 -> Bus Selector1/1
  Bus Selector1/1 -> Relational Operator/1, Switch/1  "<RadarTar2_ID_A>"
  Bus Selector1/2 -> Relational Operator/2  "<RadarTar2_ID_B>"

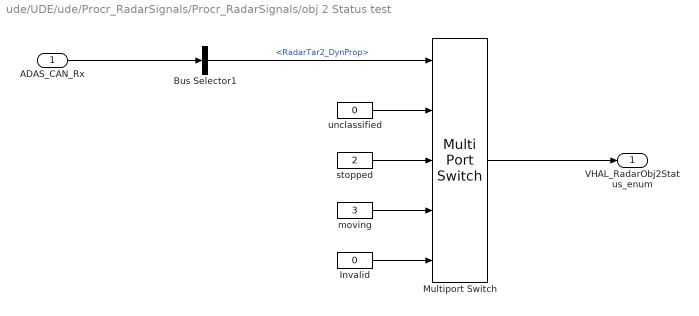
== system ude/UDE/ude/Procr_RadarSignals/Procr_RadarSignals/obj 2 Status test ==
  ADAS_CAN_Rx : Inport
  Bus Selector1 : BusSelector  OutputSignals=SENP49.RadarTar2_DynProp
  Invalid : Constant  Value=0
  Multiport Switch : MultiPortSwitch  DataPortOrder=Zero-based contiguous  Inputs=4
  moving : Constant  Value=3
  stopped : Constant  Value=2
  unclassified : Constant  Value=0
  VHAL_RadarObj2Status_enum : Outport
  wires:
  ADAS_CAN_Rx/1 -> Bus Selector1/1
  Bus Selector1/1 -> Multiport Switch/1  "<RadarTar2_DynProp>"
  unclassified/1 -> Multiport Switch/2
  stopped/1 -> Multiport Switch/3
  moving/1 -> Multiport Switch/4
  Invalid/1 -> Multiport Switch/5
  Multiport Switch/1 -> VHAL_RadarObj2Status_enum/1

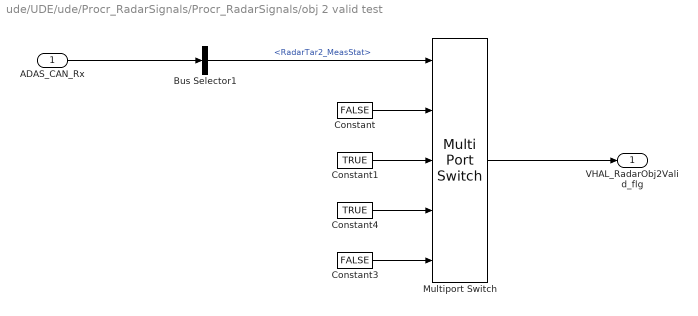
== system ude/UDE/ude/Procr_RadarSignals/Procr_RadarSignals/obj 2 valid test ==
  ADAS_CAN_Rx : Inport
  Bus Selector1 : BusSelector  OutputSignals=SENP49.RadarTar2_MeasStat
  Constant : Constant  Value=FALSE
  Constant1 : Constant  Value=TRUE
  Constant3 : Constant  Value=FALSE
  Constant4 : Constant  Value=TRUE
  Multiport Switch : MultiPortSwitch  DataPortOrder=Zero-based contiguous  Inputs=4
  VHAL_RadarObj2Valid_flg : Outport
  wires:
  ADAS_CAN_Rx/1 -> Bus Selector1/1
  Bus Selector1/1 -> Multiport Switch/1  "<RadarTar2_MeasStat>"
  Constant/1 -> Multiport Switch/2
  Constant1/1 -> Multiport Switch/3
  Constant4/1 -> Multiport Switch/4
  Constant3/1 -> Multiport Switch/5
  Multiport Switch/1 -> VHAL_RadarObj2Valid_flg/1

== system ude/UDE/ude/Procr_RadarSignals/Procr_RadarSignals/obj 2 width test ==
  VHAL_RadarObj2Valid_flg : Inport
  Constant : Constant  Value=0
  Constant1 : Constant  Value=2
  Multiport Switch : MultiPortSwitch  DataPortOrder=Zero-based contiguous  Inputs=2
  VHAL_RadarObj2Width_m : Outport
  wires:
  VHAL_RadarObj2Valid_flg/1 -> Multiport Switch/1
  Constant/1 -> Multiport Switch/2
  Constant1/1 -> Multiport Switch/3
  Multiport Switch/1 -> VHAL_RadarObj2Width_m/1

== system ude/UDE/ude/Procr_RadarSignals/Procr_RadarSignals/obj 3 ID compare ==
  ADAS_CAN_Rx : Inport
  Bus Selector1 : BusSelector  OutputSignals=SENP50.RadarTar3_ID_A,SENP51.RadarTar3_ID_B
  Constant : Constant  Value=0
  Relational Operator : RelationalOperator  Operator===  OutDataTypeStr=boolean
  Switch : Switch  Criteria=u2 ~= 0
  VHAL_RadarObj3ID_enum : Outport
  wires:
  Bus Selector1/2 -> Relational Operator/2  "<RadarTar3_ID_B>"
  Bus Selector1/1 -> Switch/1, Relational Operator/1  "<RadarTar3_ID_A>"
  ADAS_CAN_Rx/1 -> Bus Selector1/1
  Switch/1 -> VHAL_RadarObj3ID_enum/1
  Relational Operator/1 -> Switch/2
  Constant/1 -> Switch/3

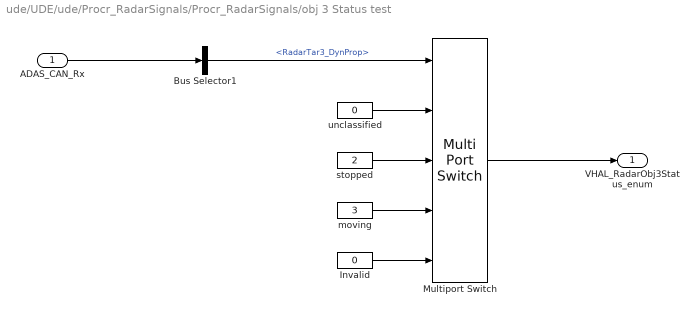
== system ude/UDE/ude/Procr_RadarSignals/Procr_RadarSignals/obj 3 Status test ==
  ADAS_CAN_Rx : Inport
  Bus Selector1 : BusSelector  OutputSignals=SENP51.RadarTar3_DynProp
  Invalid : Constant  Value=0
  Multiport Switch : MultiPortSwitch  DataPortOrder=Zero-based contiguous  Inputs=4
  moving : Constant  Value=3
  stopped : Constant  Value=2
  unclassified : Constant  Value=0
  VHAL_RadarObj3Status_enum : Outport
  wires:
  Multiport Switch/1 -> VHAL_RadarObj3Status_enum/1
  Invalid/1 -> Multiport Switch/5
  moving/1 -> Multiport Switch/4
  stopped/1 -> Multiport Switch/3
  unclassified/1 -> Multiport Switch/2
  Bus Selector1/1 -> Multiport Switch/1  "<RadarTar3_DynProp>"
  ADAS_CAN_Rx/1 -> Bus Selector1/1

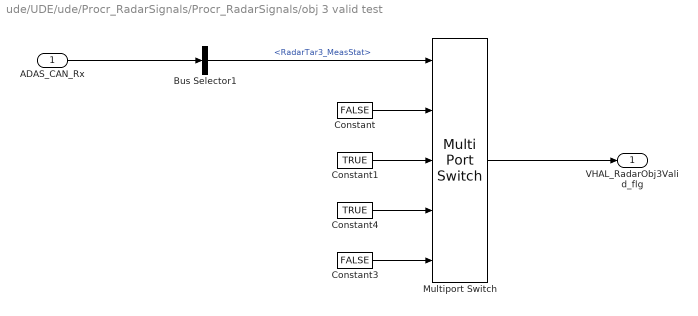
== system ude/UDE/ude/Procr_RadarSignals/Procr_RadarSignals/obj 3 valid test ==
  ADAS_CAN_Rx : Inport
  Bus Selector1 : BusSelector  OutputSignals=SENP51.RadarTar3_MeasStat
  Constant : Constant  Value=FALSE
  Constant1 : Constant  Value=TRUE
  Constant3 : Constant  Value=FALSE
  Constant4 : Constant  Value=TRUE
  Multiport Switch : MultiPortSwitch  DataPortOrder=Zero-based contiguous  Inputs=4
  VHAL_RadarObj3Valid_flg : Outport
  wires:
  Multiport Switch/1 -> VHAL_RadarObj3Valid_flg/1
  Constant3/1 -> Multiport Switch/5
  Constant4/1 -> Multiport Switch/4
  Constant1/1 -> Multiport Switch/3
  Constant/1 -> Multiport Switch/2
  Bus Selector1/1 -> Multiport Switch/1  "<RadarTar3_MeasStat>"
  ADAS_CAN_Rx/1 -> Bus Selector1/1

== system ude/UDE/ude/Procr_RadarSignals/Procr_RadarSignals/obj 3 width test ==
  VHAL_RadarObj3Valid_flg : Inport
  Constant : Constant  Value=0
  Constant1 : Constant  Value=2
  Multiport Switch : MultiPortSwitch  DataPortOrder=Zero-based contiguous  Inputs=2
  VHAL_RadarObj3Width_m : Outport
  wires:
  VHAL_RadarObj3Valid_flg/1 -> Multiport Switch/1
  Constant/1 -> Multiport Switch/2
  Constant1/1 -> Multiport Switch/3
  Multiport Switch/1 -> VHAL_RadarObj3Width_m/1

== system ude/UDE/ude/Procr_RadarSignals/Procr_RadarSignals/obj 4 ID compare ==
  ADAS_CAN_Rx : Inport
  Bus Selector1 : BusSelector  OutputSignals=SENP52.RadarTar4_ID_A,SENP53.RadarTar4_ID_B
  Constant : Constant  Value=0
  Relational Operator : RelationalOperator  Operator===  OutDataTypeStr=boolean
  Switch : Switch  Criteria=u2 ~= 0
  VHAL_RadarObj4ID_enum : Outport
  wires:
  Constant/1 -> Switch/3
  Relational Operator/1 -> Switch/2
  Switch/1 -> VHAL_RadarObj4ID_enum/1
  ADAS_CAN_Rx/1 -> Bus Selector1/1
  Bus Selector1/1 -> Relational Operator/1, Switch/1  "<RadarTar4_ID_A>"
  Bus Selector1/2 -> Relational Operator/2  "<RadarTar4_ID_B>"

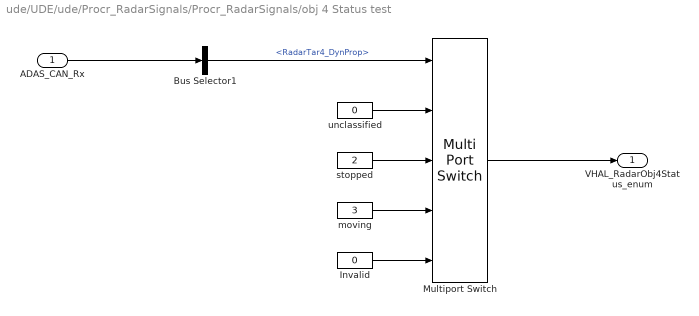
== system ude/UDE/ude/Procr_RadarSignals/Procr_RadarSignals/obj 4 Status test ==
  ADAS_CAN_Rx : Inport
  Bus Selector1 : BusSelector  OutputSignals=SENP53.RadarTar4_DynProp
  Invalid : Constant  Value=0
  Multiport Switch : MultiPortSwitch  DataPortOrder=Zero-based contiguous  Inputs=4
  moving : Constant  Value=3
  stopped : Constant  Value=2
  unclassified : Constant  Value=0
  VHAL_RadarObj4Status_enum : Outport
  wires:
  ADAS_CAN_Rx/1 -> Bus Selector1/1
  Bus Selector1/1 -> Multiport Switch/1  "<RadarTar4_DynProp>"
  unclassified/1 -> Multiport Switch/2
  stopped/1 -> Multiport Switch/3
  moving/1 -> Multiport Switch/4
  Invalid/1 -> Multiport Switch/5
  Multiport Switch/1 -> VHAL_RadarObj4Status_enum/1

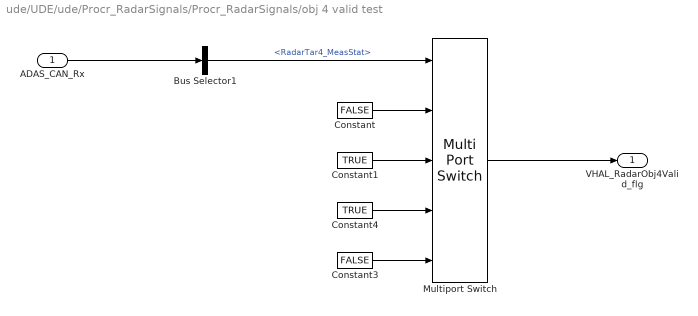
== system ude/UDE/ude/Procr_RadarSignals/Procr_RadarSignals/obj 4 valid test ==
  ADAS_CAN_Rx : Inport
  Bus Selector1 : BusSelector  OutputSignals=SENP53.RadarTar4_MeasStat
  Constant : Constant  Value=FALSE
  Constant1 : Constant  Value=TRUE
  Constant3 : Constant  Value=FALSE
  Constant4 : Constant  Value=TRUE
  Multiport Switch : MultiPortSwitch  DataPortOrder=Zero-based contiguous  Inputs=4
  VHAL_RadarObj4Valid_flg : Outport
  wires:
  ADAS_CAN_Rx/1 -> Bus Selector1/1
  Bus Selector1/1 -> Multiport Switch/1  "<RadarTar4_MeasStat>"
  Constant/1 -> Multiport Switch/2
  Constant1/1 -> Multiport Switch/3
  Constant4/1 -> Multiport Switch/4
  Constant3/1 -> Multiport Switch/5
  Multiport Switch/1 -> VHAL_RadarObj4Valid_flg/1

== system ude/UDE/ude/Procr_RadarSignals/Procr_RadarSignals/obj 4 width test ==
  VHAL_RadarObj4Valid_flg : Inport
  Constant : Constant  Value=0
  Constant1 : Constant  Value=2
  Multiport Switch : MultiPortSwitch  DataPortOrder=Zero-based contiguous  Inputs=2
  VHAL_RadarObj4Width_m : Outport
  wires:
  Multiport Switch/1 -> VHAL_RadarObj4Width_m/1
  Constant1/1 -> Multiport Switch/3
  Constant/1 -> Multiport Switch/2
  VHAL_RadarObj4Valid_flg/1 -> Multiport Switch/1

== system ude/UDE/ude/Procr_RadarSignals/Procr_RadarSignals/obj 5 ID compare ==
  ADAS_CAN_Rx : Inport
  Bus Selector1 : BusSelector  OutputSignals=SENP54.RadarTar5_ID_A,SENP55.RadarTar5_ID_B
  Constant : Constant  Value=0
  Relational Operator : RelationalOperator  Operator===  OutDataTypeStr=boolean
  Switch : Switch  Criteria=u2 ~= 0
  VHAL_RadarObj5ID_enum : Outport
  wires:
  Bus Selector1/2 -> Relational Operator/2  "<RadarTar5_ID_B>"
  Bus Selector1/1 -> Switch/1, Relational Operator/1  "<RadarTar5_ID_A>"
  ADAS_CAN_Rx/1 -> Bus Selector1/1
  Switch/1 -> VHAL_RadarObj5ID_enum/1
  Relational Operator/1 -> Switch/2
  Constant/1 -> Switch/3

== system ude/UDE/ude/Procr_RadarSignals/Procr_RadarSignals/obj 5 Status test ==
  ADAS_CAN_Rx : Inport
  Bus Selector1 : BusSelector  OutputSignals=SENP55.RadarTar5_DynProp
  Invalid : Constant  Value=0
  Multiport Switch : MultiPortSwitch  DataPortOrder=Zero-based contiguous  Inputs=4
  moving : Constant  Value=3
  stopped : Constant  Value=2
  unclassified : Constant  Value=0
  VHAL_RadarObj5Status_enum : Outport
  wires:
  Multiport Switch/1 -> VHAL_RadarObj5Status_enum/1
  Invalid/1 -> Multiport Switch/5
  moving/1 -> Multiport Switch/4
  stopped/1 -> Multiport Switch/3
  unclassified/1 -> Multiport Switch/2
  Bus Selector1/1 -> Multiport Switch/1  "<RadarTar5_DynProp>"
  ADAS_CAN_Rx/1 -> Bus Selector1/1

== system ude/UDE/ude/Procr_RadarSignals/Procr_RadarSignals/obj 5 valid test ==
  ADAS_CAN_Rx : Inport
  Bus Selector1 : BusSelector  OutputSignals=SENP55.RadarTar5_MeasStat
  Constant : Constant  Value=FALSE
  Constant1 : Constant  Value=TRUE
  Constant3 : Constant  Value=FALSE
  Constant4 : Constant  Value=TRUE
  Multiport Switch : MultiPortSwitch  DataPortOrder=Zero-based contiguous  Inputs=4
  VHAL_RadarObj5Valid_flg : Outport
  wires:
  Multiport Switch/1 -> VHAL_RadarObj5Valid_flg/1
  Constant3/1 -> Multiport Switch/5
  Constant4/1 -> Multiport Switch/4
  Constant1/1 -> Multiport Switch/3
  Constant/1 -> Multiport Switch/2
  Bus Selector1/1 -> Multiport Switch/1  "<RadarTar5_MeasStat>"
  ADAS_CAN_Rx/1 -> Bus Selector1/1

== system ude/UDE/ude/Procr_RadarSignals/Procr_RadarSignals/obj 5 width test ==
  VHAL_RadarObj5Valid_flg : Inport
  Constant : Constant  Value=0
  Constant1 : Constant  Value=2
  Multiport Switch : MultiPortSwitch  DataPortOrder=Zero-based contiguous  Inputs=2
  VHAL_RadarObj5Width_m : Outport
  wires:
  VHAL_RadarObj5Valid_flg/1 -> Multiport Switch/1
  Constant/1 -> Multiport Switch/2
  Constant1/1 -> Multiport Switch/3
  Multiport Switch/1 -> VHAL_RadarObj5Width_m/1

== system ude/UDE/ude/Procr_RadarSignals/Procr_RadarSignals/obj 6 ID compare ==
  ADAS_CAN_Rx : Inport
  Bus Selector1 : BusSelector  OutputSignals=SENP56.RadarTar6_ID_A,SENP57.RadarTar6_ID_B
  Constant : Constant  Value=0
  Relational Operator : RelationalOperator  Operator===  OutDataTypeStr=boolean
  Switch : Switch  Criteria=u2 ~= 0
  VHAL_RadarObj6ID_enum : Outport
  wires:
  Constant/1 -> Switch/3
  Relational Operator/1 -> Switch/2
  Switch/1 -> VHAL_RadarObj6ID_enum/1
  ADAS_CAN_Rx/1 -> Bus Selector1/1
  Bus Selector1/1 -> Relational Operator/1, Switch/1  "<RadarTar6_ID_A>"
  Bus Selector1/2 -> Relational Operator/2  "<RadarTar6_ID_B>"

== system ude/UDE/ude/Procr_RadarSignals/Procr_RadarSignals/obj 6 Status test ==
  ADAS_CAN_Rx : Inport
  Bus Selector1 : BusSelector  OutputSignals=SENP57.RadarTar6_DynProp
  Invalid : Constant  Value=0
  Multiport Switch : MultiPortSwitch  DataPortOrder=Zero-based contiguous  Inputs=4
  moving : Constant  Value=3
  stopped : Constant  Value=2
  unclassified : Constant  Value=0
  VHAL_RadarObj6Status_enum : Outport
  wires:
  ADAS_CAN_Rx/1 -> Bus Selector1/1
  Bus Selector1/1 -> Multiport Switch/1  "<RadarTar6_DynProp>"
  unclassified/1 -> Multiport Switch/2
  stopped/1 -> Multiport Switch/3
  moving/1 -> Multiport Switch/4
  Invalid/1 -> Multiport Switch/5
  Multiport Switch/1 -> VHAL_RadarObj6Status_enum/1

== system ude/UDE/ude/Procr_RadarSignals/Procr_RadarSignals/obj 6 valid test ==
  ADAS_CAN_Rx : Inport
  Bus Selector1 : BusSelector  OutputSignals=SENP57.RadarTar6_MeasStat
  Constant : Constant  Value=FALSE
  Constant1 : Constant  Value=TRUE
  Constant3 : Constant  Value=FALSE
  Constant4 : Constant  Value=TRUE
  Multiport Switch : MultiPortSwitch  DataPortOrder=Zero-based contiguous  Inputs=4
  VHAL_RadarObj6Valid_flg : Outport
  wires:
  ADAS_CAN_Rx/1 -> Bus Selector1/1
  Bus Selector1/1 -> Multiport Switch/1  "<RadarTar6_MeasStat>"
  Constant/1 -> Multiport Switch/2
  Constant1/1 -> Multiport Switch/3
  Constant4/1 -> Multiport Switch/4
  Constant3/1 -> Multiport Switch/5
  Multiport Switch/1 -> VHAL_RadarObj6Valid_flg/1

== system ude/UDE/ude/Procr_RadarSignals/Procr_RadarSignals/obj 6 width test ==
  VHAL_RadarObj6Valid_flg : Inport
  Constant : Constant  Value=0
  Constant1 : Constant  Value=2
  Multiport Switch : MultiPortSwitch  DataPortOrder=Zero-based contiguous  Inputs=2
  VHAL_RadarObj6Width_m : Outport
  wires:
  Multiport Switch/1 -> VHAL_RadarObj6Width_m/1
  Constant1/1 -> Multiport Switch/3
  Constant/1 -> Multiport Switch/2
  VHAL_RadarObj6Valid_flg/1 -> Multiport Switch/1
